simulink model "ha"  (R2020a)
settings: Solver=VariableStepAuto  StartTime=0.0  StopTime=10.0  RelTol=1e-3
settings Model: Creator=kishan  LastModifiedBy=kishan

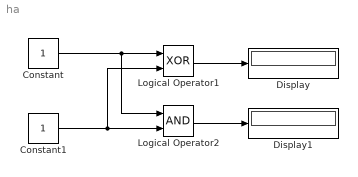
== system ha ==
  Constant : Constant
  Constant1 : Constant
  Display : Display
  Display1 : Display
  Logical Operator1 : Logic  Operator=XOR  AllPortsSameDT=off  OutDataTypeStr=boolean
  Logical Operator2 : Logic  AllPortsSameDT=off  OutDataTypeStr=boolean
  wires:
  Logical Operator1/1 -> Display/1
  Logical Operator2/1 -> Display1/1
  Constant/1 -> Logical Operator2/1, Logical Operator1/1
  Constant1/1 -> Logical Operator1/2, Logical Operator2/2
